simulink model "gtm_design_MACH"  (Simulink 7.2)
settings: Solver=ode3  SolverMode=SingleTasking  StartTime=0.0  StopTime=Inf  FixedStep=Timestep  MaxStep=0.1  MinStep=0.005  RelTol=1e-5
StopFcn:
  | MWSout=grabmws(bdroot);
  | MWSout.lastrun=datestr(now);
model workspace: external: M-Code (data not in the file)
undefined symbols (not defined in the file or in its folder): WindDir, WindSpd
libraries: simulink x2, aircraft_lib x1, Doublet_Generator_lib x1, NamedStore_lib x1
CloseFcn:
  | rtwprivate ssgensfun ModelCloseRequest gtm_design
settings Model: Creator=cox  LastModifiedBy=E183308  ExtModeAutoUpdateStatusClock=off
settings DataIOCC: MaxDataPoints=50000  SaveFormat=Structure  SaveOutput=off  SignalLogging=off
settings OptimizationCC: BooleanDataType=off  InitFltsAndDblsToZero=on
settings DebuggingCC: SaveWithParameterizedLinksMsg=none  SignalResolutionControl=TryResolveAllWithWarning  SolverPrmCheckMsg=none  InheritedTsInSrcMsg=none  MultiTaskDSMMsg=warning  MultiTaskCondExecSysMsg=none  StrictBusMsg=None
settings HardwareCC: TargetHWDeviceType=32-bit Generic
settings RTWCC: IncludeERTFirstTime=on
settings GRTTargetCC: TargetFcnLib=ansi_tfl_tmw.mat

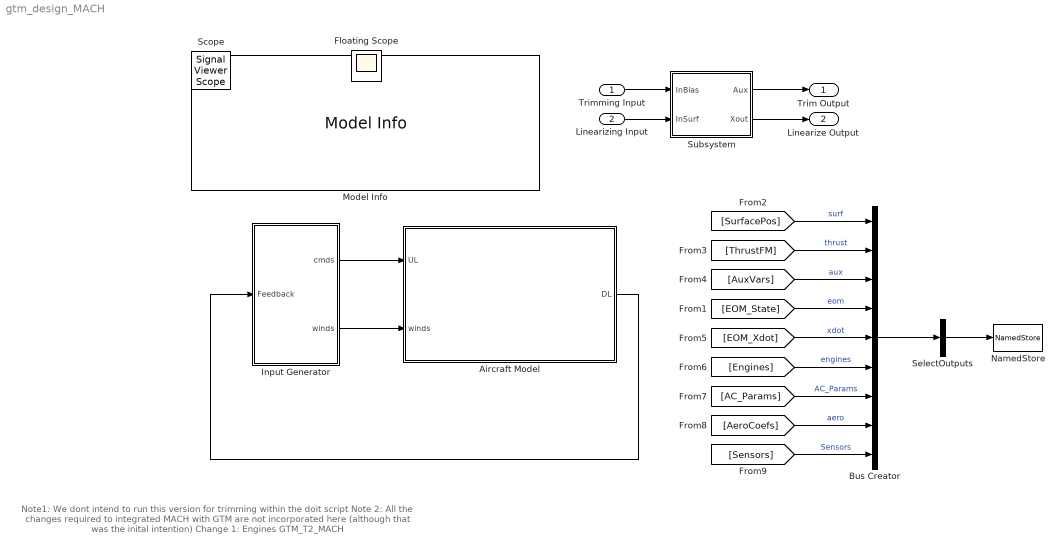
== system gtm_design_MACH ==
  note: Note1: We dont intend to run this version for trimming within the doit script
      |
      | Note 2: All the changes required to integrated MACH with GTM are not
      | incorporated here (although that was the inital intention)
      |
      | Change 1: Engines GTM_T2_MACH
  Trimming Input : Inport  PortDimensions=4  DataType=double  OutDataType=sfix(16)  OutScaling=2^0  OutDataTypeStr=double
  Linearizing Input : Inport  Port=2  PortDimensions=19  DataType=double  OutDataType=sfix(16)  OutScaling=2^0  OutDataTypeStr=double
  Aircraft Model : Subsystem  BlockChoice=GTM_T2_MACH
      link override GTM_T2/Actuators/GTM_T2/InputModification for Trim and Linearize/DriveFromTrim/MapPitchSurf/UseElevatorToTrim/Gain: Gain=[1;1;1;1;zeros(18,1)];
      link override GTM_T2/Avionics: BlockChoice=TransportDelay
      link override GTM_T2/Engines: BlockChoice=GTM_T2
      link override GTM_T2/Engines/GTM_T2/Bypass: Value=0
      link override GTM_T2/Sensors: BlockChoice=GTM_T2 gtm_design
      link override L1011_S2/Avionics: BlockChoice=Blank
      link override L1011_S2/Sensors: BlockChoice=Blank
      settings: AttributesFormatString=%<BlockChoice>  TemplateBlock=aircraft_lib/Aircraft Model  MemberBlocks=GTM_T2,GTM_T2_MACH
  Bus Creator : BusCreator  Inputs=9
  Input Generator : Subsystem
  Model Info : simulink/Model-Wide Utilities/Model Info  SystemSampleTime=-1  InitialBlockCM=none  BlockCM=none  Frame=on  DisplayStringWithTags=|  HorizontalTextAlignment=Center  LeftAlignmentValue=0.5  SourceBlockDiagram=gtm_design_MACH  TagMaxNumber=20
      | GTM Design-Simulation Model
      | Subversion Info: %<ModelVersion>
      | Last modified by %<LastModifiedBy> on %<LastModificationDate>
      | 
      | Copyright 2009
      | United States Government as represented by the 
      | Administrator of the National and Aeronautics and Space Administration.
      | 
      | No copyright is claimed in the United States under Title 17, U.S. Code.
      | All Other Rights Reserved.
  NamedStore : NamedStore_lib/NamedStore  SystemSampleTime=-1  Npts=inf  VarName=sout  expand=off
  SelectOutputs : BusSelector  OutputSignals=aux.eas,aux.alpha,aux.beta,aux.gamma  OutputAsBus=on
  Subsystem : Subsystem
  Trim Output : Outport  PortDimensions=6  DataType=double  OutDataType=sfix(16)  OutScaling=2^0  OutDataTypeStr=double
  Linearize Output : Outport  Port=2  PortDimensions=12  DataType=double  OutDataType=sfix(16)  OutScaling=2^0  OutDataTypeStr=double
  Floating Scope : Scope
      settings: Floating=on  YMin=0  YMax=7
  Scope : SignalViewerScope  IOType=viewer  RefreshTime=0.035000
  wires:
  SelectOutputs/1 -> NamedStore/1
  [SurfacePos] -> Bus Creator/1  "surf"
  Linearizing Input/1 -> Subsystem/2(InSurf)
  Subsystem/1(Aux) -> Trim Output/1
  [EOM_State] -> Bus Creator/4  "eom"
  [AuxVars] -> Bus Creator/3  "aux"
  [ThrustFM] -> Bus Creator/2  "thrust"
  Subsystem/2(Xout) -> Linearize Output/1
  [EOM_Xdot] -> Bus Creator/5  "xdot"
  [Engines] -> Bus Creator/6  "engines"
  [AC_Params] -> Bus Creator/7  "AC_Params"
  Bus Creator/1 -> SelectOutputs/1
  Aircraft Model/1(DL) -> Input Generator/1(Feedback)
  [AeroCoefs] -> Bus Creator/8  "aero"
  [Sensors] -> Bus Creator/9  "Sensors"
  Trimming Input/1 -> Subsystem/1(InBias)
  Input Generator/1(cmds) -> Aircraft Model/1(UL)
  Input Generator/2(winds) -> Aircraft Model/2(winds)

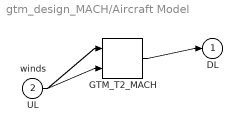
== system gtm_design_MACH/Aircraft Model ==
  UL : Inport  OutDataType=sfix(16)  OutScaling=2^0
  winds : Inport  Port=2  OutDataType=sfix(16)  OutScaling=2^0
  GTM_T2_MACH : aircraft_lib/GTM_T2_MACH  Tag=From trunk/GTMsim/gtm_model.mdl revision 162  SystemSampleTime=-1
  DL : Outport  OutDataType=sfix(16)  OutScaling=2^0
  wires:
  UL/1 -> GTM_T2_MACH/1
  winds/1 -> GTM_T2_MACH/2
  GTM_T2_MACH/1 -> DL/1

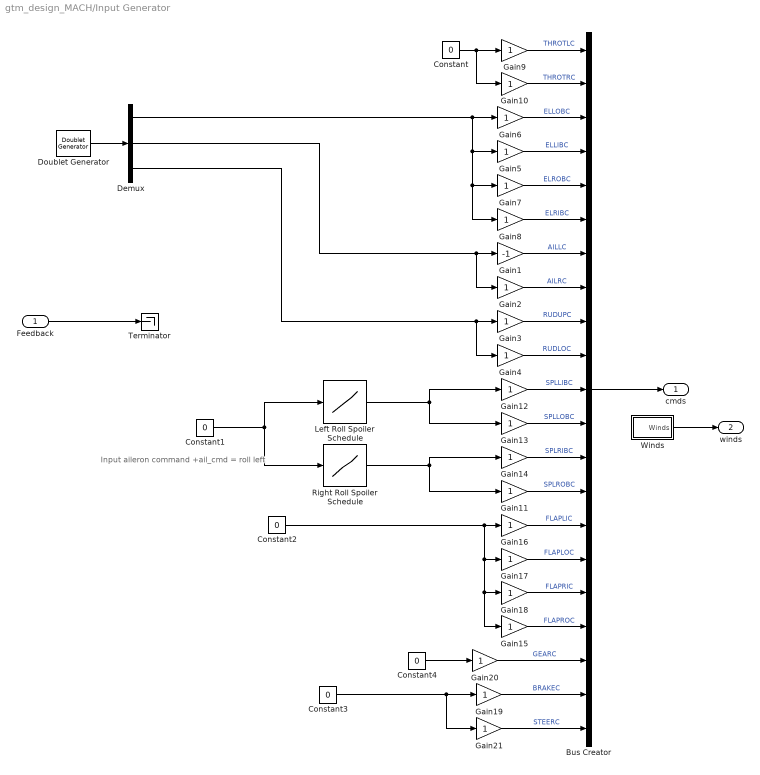
== system gtm_design_MACH/Input Generator ==
  note: Input aileron command
      | +ail_cmd = roll left
  Feedback : Inport  OutDataType=sfix(16)  OutScaling=2^0
  Bus Creator : BusCreator  Inputs=21
  Constant{,1..4} (5 alike) : Constant  Value=0  OutDataType=sfix(16)  OutScaling=2^0
  Demux : Demux  Outputs=3
  Doublet Generator : Doublet_Generator_lib/Doublet Generator  SystemSampleTime=-1  timeon=[2 12 7]  pulsewidth=[0.5 0.5 0.5]  amplitude=[0 0 0]
  Gain1 : Gain  Gain=-1  ParameterDataType=sfix(16)  ParameterScaling=2^0  OutDataType=sfix(16)  OutScaling=2^0  SaturateOnIntegerOverflow=on  OutDataTypeStr=Inherit: Same as input  ParamDataTypeStr=Inherit: Same as input
  Gain{2..21} (20 alike) : Gain  ParameterDataType=sfix(16)  ParameterScaling=2^0  OutDataType=sfix(16)  OutScaling=2^0  SaturateOnIntegerOverflow=on  OutDataTypeStr=Inherit: Same as input  ParamDataTypeStr=Inherit: Same as input
  Left Roll Spoiler Schedule : Lookup  InputValues="[-20\t-11.76\t-2.36\t0\t2.36\t11.76\t20\t]"  Table=[0 0 0 0 0 9 45]  LookUpMeth=Interpolation-Use End Values  OutDataType=sfix(16)  OutScaling=2^0
  Right Roll Spoiler Schedule : Lookup  InputValues="[-20\t-11.76\t-2.36\t0\t2.36\t11.76\t20\t]"  Table=[45 9 0 0 0 0 0]  LookUpMeth=Interpolation-Use End Values  OutDataType=sfix(16)  OutScaling=2^0
  Terminator : Terminator
  Winds : Subsystem
  cmds : Outport  OutDataType=sfix(16)  OutScaling=2^0
  winds : Outport  Port=2  OutDataType=sfix(16)  OutScaling=2^0
  wires:
  Winds/1(Winds) -> winds/1
  Constant1/1 -> Right Roll Spoiler Schedule/1, Left Roll Spoiler Schedule/1
  Right Roll Spoiler Schedule/1 -> Gain11/1, Gain14/1
  Left Roll Spoiler Schedule/1 -> Gain13/1, Gain12/1
  Gain12/1 -> Bus Creator/11  "SPLLIBC"
  Gain13/1 -> Bus Creator/12  "SPLLOBC"
  Gain14/1 -> Bus Creator/13  "SPLRIBC"
  Gain11/1 -> Bus Creator/14  "SPLROBC"
  Gain16/1 -> Bus Creator/15  "FLAPLIC"
  Gain17/1 -> Bus Creator/16  "FLAPLOC"
  Gain18/1 -> Bus Creator/17  "FLAPRIC"
  Gain15/1 -> Bus Creator/18  "FLAPROC"
  Gain9/1 -> Bus Creator/1  "THROTLC"
  Gain10/1 -> Bus Creator/2  "THROTRC"
  Gain5/1 -> Bus Creator/4  "ELLIBC"
  Gain6/1 -> Bus Creator/3  "ELLOBC"
  Gain7/1 -> Bus Creator/5  "ELROBC"
  Gain8/1 -> Bus Creator/6  "ELRIBC"
  Gain1/1 -> Bus Creator/7  "AILLC"
  Gain2/1 -> Bus Creator/8  "AILRC"
  Gain3/1 -> Bus Creator/9  "RUDUPC"
  Gain4/1 -> Bus Creator/10  "RUDLOC"
  Constant/1 -> Gain10/1, Gain9/1
  Constant2/1 -> Gain16/1, Gain17/1, Gain18/1, Gain15/1
  Doublet Generator/1 -> Demux/1
  Demux/2 -> Gain1/1, Gain2/1
  Demux/3 -> Gain3/1, Gain4/1
  Gain19/1 -> Bus Creator/20  "BRAKEC"
  Constant4/1 -> Gain20/1
  Constant3/1 -> Gain19/1, Gain21/1
  Demux/1 -> Gain6/1, Gain5/1, Gain7/1, Gain8/1
  Bus Creator/1 -> cmds/1
  Gain20/1 -> Bus Creator/19  "GEARC"
  Gain21/1 -> Bus Creator/21  "STEERC"
  Feedback/1 -> Terminator/1

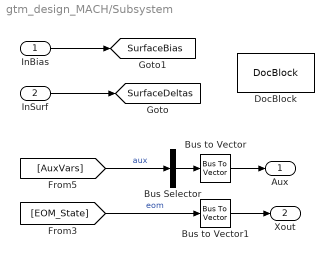
== system gtm_design_MACH/Subsystem ==
  InBias : Inport  OutDataType=sfix(16)  OutScaling=2^0
  InSurf : Inport  Port=2  OutDataType=sfix(16)  OutScaling=2^0
  Bus Selector : BusSelector  OutputSignals=eas,tas,alpha,beta,gamma,gndtrack  OutputAsBus=on
  Bus to Vector : BusToVector
  Bus to Vector1 : BusToVector
  DocBlock : simulink/Model-Wide Utilities/DocBlock  SystemSampleTime=-1  DocumentType=Text
      content=|
      | Inputs and Outputs selected here have a specific ordering.
      |
      |
      |
      | Do not change this without also changing output channel ordering in associated linmodel.m and
      | trimgtm.m functions
  Aux : Outport  OutDataType=sfix(16)  OutScaling=2^0
  Xout : Outport  Port=2  OutDataType=sfix(16)  OutScaling=2^0
  tag scope: SurfaceBias=global, SurfaceDeltas=global
  wires:
  [AuxVars] -> Bus Selector/1  "aux"
  [EOM_State] -> Bus to Vector1/1  "eom"
  Bus Selector/1 -> Bus to Vector/1
  InSurf/1 -> [SurfaceDeltas]
  Bus to Vector/1 -> Aux/1
  Bus to Vector1/1 -> Xout/1
  InBias/1 -> [SurfaceBias]

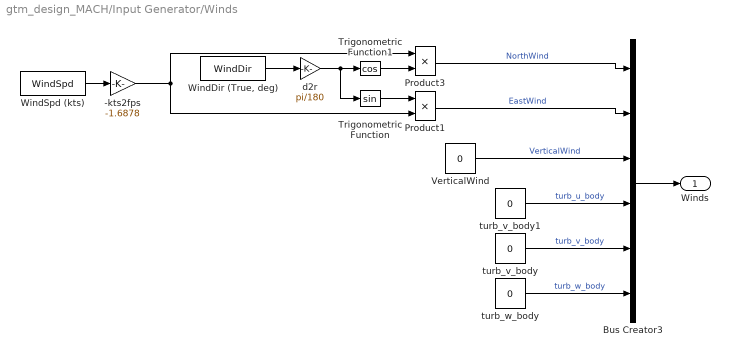
== system gtm_design_MACH/Input Generator/Winds ==
  -kts2fps : Gain  Gain=-1.6878  ParameterDataType=sfix(16)  ParameterScaling=2^0  OutDataType=sfix(16)  OutScaling=2^0  SaturateOnIntegerOverflow=on  OutDataTypeStr=Inherit: Same as input  ParamDataTypeStr=Inherit: Same as input
  Bus Creator3 : BusCreator  Inputs=6
  Product1 : Product  Inputs=**  OutDataType=sfix(16)  OutScaling=2^0  SaturateOnIntegerOverflow=on  InputSameDT=on  OutDataTypeStr=Inherit: Same as first input
  Product3 : Product  Inputs=**  OutDataType=sfix(16)  OutScaling=2^0  SaturateOnIntegerOverflow=on  InputSameDT=on  OutDataTypeStr=Inherit: Same as first input
  Trigonometric Function : Trigonometry
  Trigonometric Function1 : Trigonometry  Operator=cos
  VerticalWind : Constant  Value=0  OutDataType=sfix(16)  OutScaling=2^0
  "WindDir (True, deg)" : Constant  Value=WindDir  OutDataType=sfix(16)  OutScaling=2^0
  WindSpd (kts) : Constant  Value=WindSpd  OutDataType=sfix(16)  OutScaling=2^0
  d2r : Gain  Gain=pi/180  ParameterDataType=sfix(16)  ParameterScaling=2^0  OutDataType=sfix(16)  OutScaling=2^0  SaturateOnIntegerOverflow=on  OutDataTypeStr=Inherit: Same as input  ParamDataTypeStr=Inherit: Same as input
  turb_v_body : Constant  Value=0  OutDataType=sfix(16)  OutScaling=2^0
  turb_v_body1 : Constant  Value=0  OutDataType=sfix(16)  OutScaling=2^0
  turb_w_body : Constant  Value=0  OutDataType=sfix(16)  OutScaling=2^0
  Winds : Outport  OutDataType=sfix(16)  OutScaling=2^0
  wires:
  turb_w_body/1 -> Bus Creator3/6  "turb_w_body"
  turb_v_body/1 -> Bus Creator3/5  "turb_v_body"
  turb_v_body1/1 -> Bus Creator3/4  "turb_u_body"
  -kts2fps/1 -> Product1/2, Product3/1
  WindSpd (kts)/1 -> -kts2fps/1
  "WindDir (True, deg)"/1 -> d2r/1
  d2r/1 -> Trigonometric Function1/1, Trigonometric Function/1
  Trigonometric Function1/1 -> Product3/2
  Trigonometric Function/1 -> Product1/1
  Bus Creator3/1 -> Winds/1
  VerticalWind/1 -> Bus Creator3/3  "VerticalWind"
  Product1/1 -> Bus Creator3/2  "EastWind"
  Product3/1 -> Bus Creator3/1  "NorthWind"
